simulink library "CryoDetLibCMB"  (R2016b)
settings: Solver=VariableStepAuto  StartTime=0.0  StopTime=10.0  RelTol=1e-3
undefined symbols (not defined in the file): A, B, C, D, Fadc, Fclk, PCIN, xlipgetpartsetting
libraries: xbsIndex_r4 x640, CryoDetLibCMB x81, CryoDetLib x2, simulink x1
(part 1 of 12)
settings Model: Creator=ssmith  LastModifiedBy=mdewart

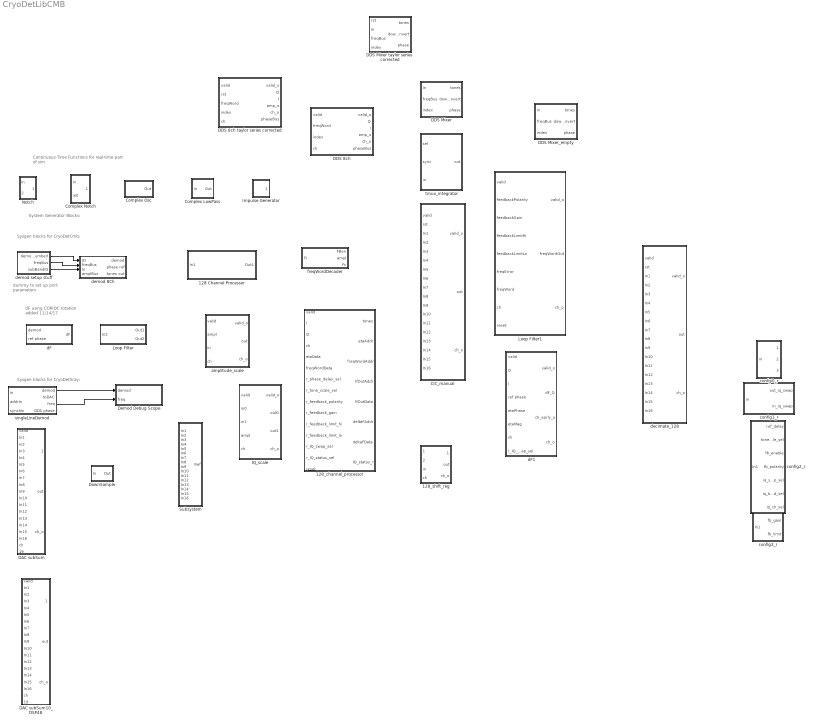
== system CryoDetLibCMB ==
  note: dummy to set up port parameters
  note: Sysgen blocks for CryoDetXray:
  note: Continuous-Time Functions
      | for real-time part of sim
  note: System Generator Blocks:
  note: Sysgen blocks for CryoDetCmb:
  note: dF using CORIDC rotation
      | added 11/14/17
  128 Channel Processor : Subsystem
  128_channel_processor : Subsystem
  128_shift_reg : Subsystem
  CIC_manual : Subsystem  mask{n_bit=30, b_pt=15}
      mask prompts: n_bit "Number of bits"; b_pt "Binary point"
  Complex LowPass : Subsystem  mask{num=0, den=0}
  Complex Notch : Subsystem  mask(Complex Notch Filter){Q=10, depth=1, Q1=10, depth1=1, Q2=10, depth2=1}
      mask help: Specify w0, Q, and notch depth (1 is max depth, 0 is no notch)
      mask init:
      | Q1 = Q
      | depth1 = depth
      | Q2 = Q
      | depth2 = depth
      mask TypeOptions Q1: Notch1/Q
      mask TypeOptions depth1: Notch1/depth
      mask TypeOptions Q2: Notch2/Q
      mask TypeOptions depth2: Notch2/depth
  Complex Osc : Subsystem  mask{Freq=40e6, Ampl=0.2}
  DAC subSum : Subsystem
  DAC subSum10_DSP48 : Subsystem  VariantControl=Variant1
  DDS 8ch : Subsystem
  DDS 8ch taylor series corrected : Subsystem
  DDS Mixer : Subsystem
  DDS Mixer taylor series corrected : Subsystem
  DDS Mixer_empty : Subsystem
  Demod Debug Scope : Subsystem
  DownSample : Subsystem
  IQ_scale : Subsystem
  Impulse Generator : Subsystem  mask(Impulse Generator){Impulse=0, width=0, Period=0, delay=0}
      mask help:
      | Generate an psuedo-impulse via a rectangular pulse of amplitude given impulse/width so time intagral is impulse
      | repeating at period given by parameter Period starting at time "delay"
  Loop Filter : Subsystem
  Loop Filter1 : Subsystem
  Notch : Subsystem  mask(Notch filter){Q=10, depth=1}
      mask help:
      | Continuous-time notch filter acting in input with input parameters:
      | w0	center frequency
      | Q	center frequency/bandwidth
      | depth	depth of notch: 0==> no notch, 1 ==> deep notch
  Subsystem : Subsystem
  amplitude_scale : Subsystem
  confgi0_r : Subsystem
  config1_r : Subsystem
  config2_r : Subsystem
  config3_r : Subsystem
  dF : Subsystem
  dF1 : Subsystem
  decimate_128 : Subsystem
  demod 8Ch : Subsystem
  demod setup stuff : Subsystem
  freqWordDecoder : Subsystem
  singleLineDemod : Subsystem
  tmux_integrator : Subsystem  mask{n_bit=18, b_pt=0}
      mask prompts: n_bit "Number of bits"; b_pt "Binary point"
  wires:
  singleLineDemod/3(freq) -> Demod Debug Scope/2(freq)
  singleLineDemod/1(demod) -> Demod Debug Scope/1(demod)
  demod setup stuff/3(subBandIQ) -> demod 8Ch/3(In)
  demod setup stuff/1(demod numberl) -> demod 8Ch/1(ID)
  demod setup stuff/2(freqBus) -> demod 8Ch/2(freqBus)

== system CryoDetLibCMB/128 Channel Processor ==
  note: 128 Channel Processor
      | Contains baeband tone generator
      | demodulator
      | resonator frequency error estimator
      | loop filter
  In1 : Inport
  128 Channel Demodulator : Subsystem
  Loop Filter : Subsystem
  dF : Subsystem
  Out1 : Outport
  wires:
  In1/1 -> 128 Channel Demodulator/1(in)
  dF/1(Out1) -> Loop Filter/1(In1)
  128 Channel Demodulator/1(demod) -> dF/1(demod in)
  Loop Filter/1(Out1) -> 128 Channel Demodulator/2(freqBus)
  128 Channel Demodulator/2(phase ref out) -> dF/2(phase ref in)

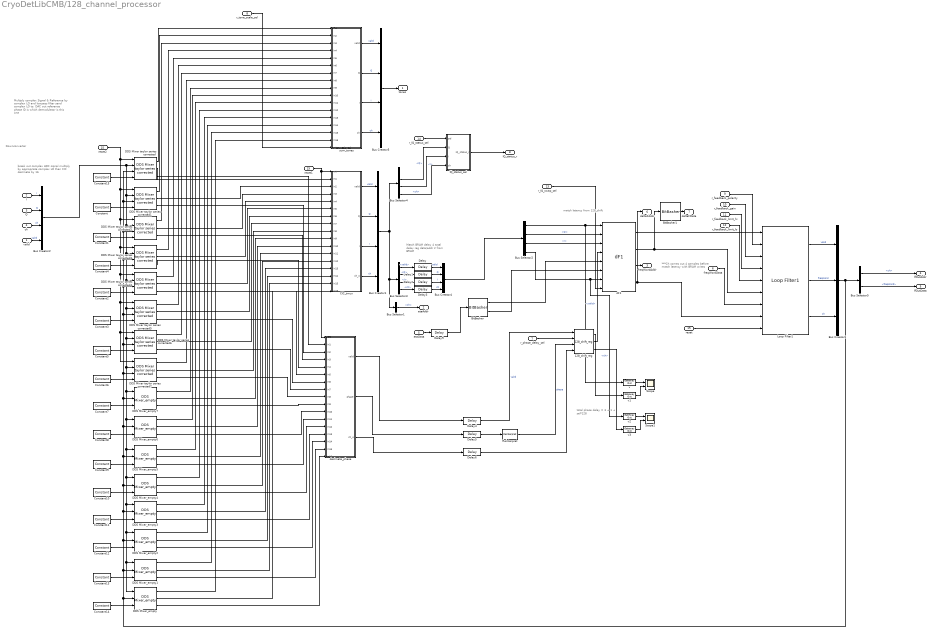
== system CryoDetLibCMB/128_channel_processor ==
  note: ***Ch comes out 4 samples before
      | match latency with BRAM writes
  note: total phase delay =
      | 3 + 1 + sel*128
  note: match latency from 128_shift
  note: Match BRAM delay
      | 4 total delay
      |    reg data/addr
      |    2 from BRAM
  note: break out complex ADC signal
      | multiply by appropriate complex LO
      | then CIC decimate by 16
  note: Multiply complex Signal & Reference
      | by complex LO and lowpass filter
      | send complex LO to:
      | 	DAC out
      | 	reference phase
      | ID is which demodulator is this one
  note: Downconverter
  valid : Inport
  I : Inport  Port=2
  Q : Inport  Port=3
  ch : Inport  Port=4
  etaData : Inport  Port=5
  freqWordData : Inport  Port=6
  r_phase_delay_sel : Inport  Port=7
  r_tone_scale_sel : Inport  Port=8
  r_feedback_polarity : Inport  Port=9
  r_feedback_gain : Inport  Port=10
  r_feedback_limit_hi : Inport  Port=11
  r_feedback_limit_lo : Inport  Port=12
  r_IQ_swap_sel : Inport  Port=13
  r_IQ_status_sel : Inport  Port=14
  reset : Inport  Port=15
  128_shift_reg : CryoDetLibCMB/128_shift_reg
  BitBasher : xbsIndex_r4/BitBasher  bitexpr=|  display_expr=off  sr_1=etaPhase  arith_type1="Signed  (2's comp)"  bin_pt1=15  sr_2=etaMag  arith_type2="Signed  (2's comp)"  bin_pt2=10  sr_3=3  arith_type3=Unsigned  bin_pt3=0  sr_4=4  arith_type4=Unsigned  bin_pt4=0  dbl_ovrd=off  block_type=bitbasher
      | etaPhase = {in[31:16]}
      | etaMag = {in[15:0]}
  BitBasher1 : xbsIndex_r4/BitBasher  bitexpr=deltaF = {8'b0, in[23:0]}  display_expr=off  sr_1=deltaF  arith_type1="Signed  (2's comp)"  bin_pt1=15  sr_2=etaMag  arith_type2="Signed  (2's comp)"  bin_pt2=10  sr_3=3  arith_type3=Unsigned  bin_pt3=0  sr_4=4  arith_type4=Unsigned  bin_pt4=0  dbl_ovrd=off  block_type=bitbasher
  Bus Creator{1..2,4..5} (4 alike) : BusCreator  Inputs=4
  Bus Creator3 : BusCreator  Inputs=3
  Bus Selector1 : BusSelector  OutputSignals=ch
  Bus Selector2 : BusSelector  OutputSignals=valid,Q,I,ch
  Bus Selector3 : BusSelector  OutputSignals=valid,Q,I,ch
  Bus Selector4 : BusSelector  OutputSignals=valid,Q,I,ch
  Bus Selector5 : BusSelector  OutputSignals=ch,freqWord
  CIC_tmux : Subsystem
  Constant : xbsIndex_r4/Constant  const=1  gui_display_data_type=Fixed-point  arith_type=Unsigned  n_bits=4  bin_pt=0  preci_type=Single  exp_width=8  frac_width=24  explicit_period=off  period=1  equ=P=C  opselect=C  inp2=PCIN>>17  opr=+  inp1=P  carry=CIN  dbl_ovrd=off  block_type=constant
  Constant1 : xbsIndex_r4/Constant  const=2  gui_display_data_type=Fixed-point  arith_type=Unsigned  n_bits=4  bin_pt=0  preci_type=Single  exp_width=8  frac_width=24  explicit_period=off  period=1  equ=P=C  opselect=C  inp2=PCIN>>17  opr=+  inp1=P  carry=CIN  dbl_ovrd=off  block_type=constant
  Constant10 : xbsIndex_r4/Constant  const=11  gui_display_data_type=Fixed-point  arith_type=Unsigned  n_bits=4  bin_pt=0  preci_type=Single  exp_width=8  frac_width=24  explicit_period=off  period=1  equ=P=C  opselect=C  inp2=PCIN>>17  opr=+  inp1=P  carry=CIN  dbl_ovrd=off  block_type=constant
  Constant11 : xbsIndex_r4/Constant  const=12  gui_display_data_type=Fixed-point  arith_type=Unsigned  n_bits=4  bin_pt=0  preci_type=Single  exp_width=8  frac_width=24  explicit_period=off  period=1  equ=P=C  opselect=C  inp2=PCIN>>17  opr=+  inp1=P  carry=CIN  dbl_ovrd=off  block_type=constant
  Constant12 : xbsIndex_r4/Constant  const=13  gui_display_data_type=Fixed-point  arith_type=Unsigned  n_bits=4  bin_pt=0  preci_type=Single  exp_width=8  frac_width=24  explicit_period=off  period=1  equ=P=C  opselect=C  inp2=PCIN>>17  opr=+  inp1=P  carry=CIN  dbl_ovrd=off  block_type=constant
  Constant13 : xbsIndex_r4/Constant  const=14  gui_display_data_type=Fixed-point  arith_type=Unsigned  n_bits=4  bin_pt=0  preci_type=Single  exp_width=8  frac_width=24  explicit_period=off  period=1  equ=P=C  opselect=C  inp2=PCIN>>17  opr=+  inp1=P  carry=CIN  dbl_ovrd=off  block_type=constant
  Constant14 : xbsIndex_r4/Constant  const=15  gui_display_data_type=Fixed-point  arith_type=Unsigned  n_bits=4  bin_pt=0  preci_type=Single  exp_width=8  frac_width=24  explicit_period=off  period=1  equ=P=C  opselect=C  inp2=PCIN>>17  opr=+  inp1=P  carry=CIN  dbl_ovrd=off  block_type=constant
  Constant15 : xbsIndex_r4/Constant  const=0  gui_display_data_type=Fixed-point  arith_type=Unsigned  n_bits=4  bin_pt=0  preci_type=Single  exp_width=8  frac_width=24  explicit_period=off  period=1  equ=P=C  opselect=C  inp2=PCIN>>17  opr=+  inp1=P  carry=CIN  dbl_ovrd=off  block_type=constant
  Constant2 : xbsIndex_r4/Constant  const=4  gui_display_data_type=Fixed-point  arith_type=Unsigned  n_bits=4  bin_pt=0  preci_type=Single  exp_width=8  frac_width=24  explicit_period=off  period=1  equ=P=C  opselect=C  inp2=PCIN>>17  opr=+  inp1=P  carry=CIN  dbl_ovrd=off  block_type=constant
  Constant3 : xbsIndex_r4/Constant  const=5  gui_display_data_type=Fixed-point  arith_type=Unsigned  n_bits=4  bin_pt=0  preci_type=Single  exp_width=8  frac_width=24  explicit_period=off  period=1  equ=P=C  opselect=C  inp2=PCIN>>17  opr=+  inp1=P  carry=CIN  dbl_ovrd=off  block_type=constant
  Constant4 : xbsIndex_r4/Constant  const=3  gui_display_data_type=Fixed-point  arith_type=Unsigned  n_bits=4  bin_pt=0  preci_type=Single  exp_width=8  frac_width=24  explicit_period=off  period=1  equ=P=C  opselect=C  inp2=PCIN>>17  opr=+  inp1=P  carry=CIN  dbl_ovrd=off  block_type=constant
  Constant5 : xbsIndex_r4/Constant  const=6  gui_display_data_type=Fixed-point  arith_type=Unsigned  n_bits=4  bin_pt=0  preci_type=Single  exp_width=8  frac_width=24  explicit_period=off  period=1  equ=P=C  opselect=C  inp2=PCIN>>17  opr=+  inp1=P  carry=CIN  dbl_ovrd=off  block_type=constant
  Constant6 : xbsIndex_r4/Constant  const=7  gui_display_data_type=Fixed-point  arith_type=Unsigned  n_bits=4  bin_pt=0  preci_type=Single  exp_width=8  frac_width=24  explicit_period=off  period=1  equ=P=C  opselect=C  inp2=PCIN>>17  opr=+  inp1=P  carry=CIN  dbl_ovrd=off  block_type=constant
  Constant7 : xbsIndex_r4/Constant  const=8  gui_display_data_type=Fixed-point  arith_type=Unsigned  n_bits=4  bin_pt=0  preci_type=Single  exp_width=8  frac_width=24  explicit_period=off  period=1  equ=P=C  opselect=C  inp2=PCIN>>17  opr=+  inp1=P  carry=CIN  dbl_ovrd=off  block_type=constant
  Constant8 : xbsIndex_r4/Constant  const=9  gui_display_data_type=Fixed-point  arith_type=Unsigned  n_bits=4  bin_pt=0  preci_type=Single  exp_width=8  frac_width=24  explicit_period=off  period=1  equ=P=C  opselect=C  inp2=PCIN>>17  opr=+  inp1=P  carry=CIN  dbl_ovrd=off  block_type=constant
  Constant9 : xbsIndex_r4/Constant  const=10  gui_display_data_type=Fixed-point  arith_type=Unsigned  n_bits=4  bin_pt=0  preci_type=Single  exp_width=8  frac_width=24  explicit_period=off  period=1  equ=P=C  opselect=C  inp2=PCIN>>17  opr=+  inp1=P  carry=CIN  dbl_ovrd=off  block_type=constant
  DDS Mixer taylor series corrected : CryoDetLibCMB/DDS Mixer taylor series corrected
      link override DDS 8ch taylor series corrected/BitBasher5: bitexpr=phase = {in[23:8]}  display_expr=off  sr_1=phase  arith_type1="Signed  (2's comp)"  bin_pt1=15  sr_2=amp  arith_type2=Unsigned  bin_pt2=0  sr_3=3  arith_type3=Unsigned  bin_pt3=0  sr_4=4  arith_type4=Unsigned  bin_pt4=0  dbl_ovrd=off
      link override DDS 8ch taylor series corrected/BitBasher5: infoedit=Allows extraction, concatenation and augmentation of bits
  DDS Mixer taylor series corrected{1..7} (7 alike) : CryoDetLibCMB/DDS Mixer taylor series corrected
  DDS Mixer_empty{,1..7} (8 alike) : CryoDetLibCMB/DDS Mixer_empty
  Delay{,1..3} (4 alike) : xbsIndex_r4/Delay  rst=off  infoeditControl=Selection of Reset will increase slice count due to use of real FFs and instead of SRLs  en=off  latency=5  reg_retiming=off  dbl_ovrd=off  block_type=delay
  Delay4 : xbsIndex_r4/Delay  rst=off  infoeditControl=Selection of Reset will increase slice count due to use of real FFs and instead of SRLs  en=off  latency=12  reg_retiming=off  dbl_ovrd=off  block_type=delay
  Delay5 : xbsIndex_r4/Delay  rst=off  infoeditControl=Selection of Reset will increase slice count due to use of real FFs and instead of SRLs  en=off  latency=12  reg_retiming=off  dbl_ovrd=off  block_type=delay
  Delay6 : xbsIndex_r4/Delay  rst=off  infoeditControl=Selection of Reset will increase slice count due to use of real FFs and instead of SRLs  en=off  latency=12  reg_retiming=off  dbl_ovrd=off  block_type=delay
  Delay9 : xbsIndex_r4/Delay  rst=off  infoeditControl=Selection of Reset will increase slice count due to use of real FFs and instead of SRLs  en=off  latency=1  reg_retiming=off  dbl_ovrd=off  block_type=delay
  IQ_status_sel : Subsystem
  Loop Filter1 : CryoDetLibCMB/Loop Filter1
  Reinterpret : xbsIndex_r4/Reinterpret  force_arith_type=on  arith_type="Signed  (2's comp)"  force_bin_pt=on  bin_pt=15  block_type=reinterpret
  Scope : Scope  NumInputPorts=2
  Scope1 : Scope  NumInputPorts=2
  dF1 : CryoDetLibCMB/dF1
  decimate_phase : Subsystem
  reset1 : InportShadow  Port=15
  reset2 : InportShadow  Port=15
  sum_tones : Subsystem
  v{,1..3} (4 alike) : xbsIndex_r4/Gateway Out  inherit_from_input=off  hdl_port=off  rows=1  columns=1  UseAsDAC=off  DACChannel='1'  interface=None  automatic_assignment=on  address_offset=hex2dec('00')  intf_name=''  intf_description=''  timing_constraint=None  locs_specified=off  LOCs={}  io_standard={}  block_type=gatewayout
  tones : Outport
  etaAddr : Outport  Port=2
  freqWordAddr : Outport  Port=3
  lfOutAddr : Outport  Port=4
  lfOutData : Outport  Port=5
  deltaFAddr : Outport  Port=6
  deltaFData : Outport  Port=7
  IQ_status_r : Outport  Port=8
  wires:
  reset2/1 -> DDS Mixer taylor series corrected2/1, DDS Mixer taylor series corrected3/1, DDS Mixer taylor series corrected4/1, DDS Mixer taylor series corrected5/1, DDS Mixer taylor series corrected6/1, DDS Mixer taylor series corrected7/1, DDS Mixer taylor series corrected1/1, DDS Mixer taylor series corrected/1
  Bus Creator3/1 -> DDS Mixer_empty/2, DDS Mixer_empty1/2, DDS Mixer_empty2/2, DDS Mixer_empty3/2, DDS Mixer_empty4/2, DDS Mixer_empty5/2, DDS Mixer taylor series corrected/3, DDS Mixer taylor series corrected1/3, DDS Mixer taylor series corrected2/3, DDS Mixer taylor series corrected3/3, DDS Mixer taylor series corrected4/3, DDS Mixer taylor series corrected5/3, DDS Mixer taylor series corrected6/3, DDS Mixer taylor series corrected7/3, DDS Mixer_empty7/2, DDS Mixer_empty6/2, Bus Selector5/1
  Constant6/1 -> DDS Mixer taylor series corrected7/4
  Constant5/1 -> DDS Mixer taylor series corrected6/4
  Constant3/1 -> DDS Mixer taylor series corrected5/4
  Constant2/1 -> DDS Mixer taylor series corrected4/4
  Constant4/1 -> DDS Mixer taylor series corrected3/4
  Constant1/1 -> DDS Mixer taylor series corrected2/4
  Constant/1 -> DDS Mixer taylor series corrected1/4
  Constant15/1 -> DDS Mixer taylor series corrected/4
  reset1/1 -> CIC_tmux/1(rst), decimate_phase/1(rst)
  Delay6/1 -> 128_shift_reg/4
  Delay9/1 -> BitBasher/1
  IQ_status_sel/1(IQ_status_r) -> IQ_status_r/1
  r_IQ_status_sel/1 -> IQ_status_sel/1(sel)
  Bus Selector4/4 -> IQ_status_sel/4(ch)  "<ch>"
  Bus Selector4/3 -> IQ_status_sel/3(I)  "<I>"
  Bus Selector4/2 -> IQ_status_sel/2(Q)  "<Q>"
  r_IQ_swap_sel/1 -> dF1/8
  128_shift_reg/3 -> v3/1
  v3/1 -> Scope1/2
  v2/1 -> Scope1/1
  128_shift_reg/1 -> v1/1
  v1/1 -> Scope/2
  v/1 -> Scope/1
  DDS Mixer taylor series corrected/2 -> CIC_tmux/2(In1)
  DDS Mixer taylor series corrected1/2 -> CIC_tmux/3(In2)
  DDS Mixer taylor series corrected2/2 -> CIC_tmux/4(In3)
  DDS Mixer taylor series corrected3/2 -> CIC_tmux/5(In4)
  DDS Mixer taylor series corrected4/2 -> CIC_tmux/6(In5)
  DDS Mixer taylor series corrected5/2 -> CIC_tmux/7(In6)
  DDS Mixer taylor series corrected6/2 -> CIC_tmux/8(In7)
  DDS Mixer taylor series corrected7/2 -> CIC_tmux/9(In8)
  DDS Mixer_empty7/2 -> CIC_tmux/10(In9)
  DDS Mixer_empty6/2 -> CIC_tmux/11(In10)
  DDS Mixer_empty5/2 -> CIC_tmux/12(In11)
  DDS Mixer_empty4/2 -> CIC_tmux/13(In12)
  DDS Mixer_empty3/2 -> CIC_tmux/14(In13)
  DDS Mixer_empty2/2 -> CIC_tmux/15(In14)
  DDS Mixer_empty1/2 -> CIC_tmux/16(In15)
  DDS Mixer_empty/2 -> CIC_tmux/17(In16)
  Bus Creator2/1 -> DDS Mixer_empty5/1, DDS Mixer_empty4/1, DDS Mixer_empty3/1, DDS Mixer_empty2/1, DDS Mixer_empty1/1, DDS Mixer_empty/1, DDS Mixer_empty6/1, DDS Mixer_empty7/1, DDS Mixer taylor series corrected7/2, DDS Mixer taylor series corrected6/2, DDS Mixer taylor series corrected5/2, DDS Mixer taylor series corrected4/2, DDS Mixer taylor series corrected3/2, DDS Mixer taylor series corrected2/2, DDS Mixer taylor series corrected1/2, DDS Mixer taylor series corrected/2
  Constant14/1 -> DDS Mixer_empty/3
  Constant13/1 -> DDS Mixer_empty1/3
  Constant12/1 -> DDS Mixer_empty2/3
  Constant11/1 -> DDS Mixer_empty3/3
  Constant10/1 -> DDS Mixer_empty4/3
  Constant9/1 -> DDS Mixer_empty5/3
  Constant8/1 -> DDS Mixer_empty6/3
  Constant7/1 -> DDS Mixer_empty7/3
  DDS Mixer taylor series corrected/1 -> sum_tones/1(In1)
  DDS Mixer taylor series corrected1/1 -> sum_tones/2(In2)
  DDS Mixer taylor series corrected2/1 -> sum_tones/3(In3)
  DDS Mixer taylor series corrected3/1 -> sum_tones/4(In4)
  DDS Mixer taylor series corrected4/1 -> sum_tones/5(In5)
  DDS Mixer taylor series corrected5/1 -> sum_tones/6(In6)
  DDS Mixer taylor series corrected6/1 -> sum_tones/7(In7)
  DDS Mixer taylor series corrected7/1 -> sum_tones/8(In8)
  DDS Mixer_empty7/1 -> sum_tones/9(In9)
  DDS Mixer_empty6/1 -> sum_tones/10(In10)
  DDS Mixer_empty5/1 -> sum_tones/11(In11)
  DDS Mixer_empty4/1 -> sum_tones/12(In12)
  DDS Mixer_empty3/1 -> sum_tones/13(In13)
  DDS Mixer_empty2/1 -> sum_tones/14(In14)
  DDS Mixer_empty1/1 -> sum_tones/15(In15)
  DDS Mixer_empty/1 -> sum_tones/16(In16)
  I/1 -> Bus Creator2/1  "I"
  Q/1 -> Bus Creator2/2  "Q"
  ch/1 -> Bus Creator2/3  "ch"
  valid/1 -> Bus Creator2/4  "valid"
  Bus Creator1/1 -> Bus Selector4/1, Bus Selector3/1, Bus Selector1/1
  Bus Selector1/1 -> etaAddr/1  "<ch>"
  Delay/1 -> Bus Creator4/1  "valid"
  Delay1/1 -> Bus Creator4/2  "Q"
  Delay2/1 -> Bus Creator4/3  "I"
  Delay3/1 -> Bus Creator4/4  "ch"
  etaData/1 -> Delay9/1
  Bus Creator4/1 -> Bus Selector2/1
  BitBasher1/1 -> deltaFData/1
  CIC_tmux/1(valid) -> Bus Creator1/1  "valid"
  CIC_tmux/2(Q) -> Bus Creator1/2  "Q"
  CIC_tmux/3(I) -> Bus Creator1/3  "I"
  CIC_tmux/4(ch_o) -> Bus Creator1/4  "ch"
  Bus Selector3/1 -> Delay/1  "<valid>"
  Bus Selector3/2 -> Delay1/1  "<Q>"
  Bus Selector3/3 -> Delay2/1  "<I>"
  Bus Selector3/4 -> Delay3/1  "<ch>"
  sum_tones/3(I) -> Bus Creator5/3  "I"
  sum_tones/2(Q) -> Bus Creator5/2  "Q"
  sum_tones/4(ch) -> Bus Creator5/4  "ch"
  sum_tones/1(valid) -> Bus Creator5/1  "valid"
  Bus Creator5/1 -> tones/1
  Bus Selector2/1 -> dF1/1, v/1  "<valid>"
  Bus Selector2/2 -> dF1/2  "<Q>"
  Bus Selector2/3 -> dF1/3  "<I>"
  Bus Selector2/4 -> dF1/7, v2/1  "<ch>"
  128_shift_reg/2 -> dF1/4
  dF1/1 -> Loop Filter1/1
  Loop Filter1/1 -> Bus Creator3/1  "valid"
  Bus Selector5/2 -> lfOutData/1  "<freqWord>"
  Bus Selector5/1 -> lfOutAddr/1  "<ch>"
  r_phase_delay_sel/1 -> 128_shift_reg/2
  r_feedback_limit_hi/1 -> Loop Filter1/4
  r_feedback_gain/1 -> Loop Filter1/3
  r_feedback_polarity/1 -> Loop Filter1/2
  r_tone_scale_sel/1 -> sum_tones/17(r_tone_scale_sel)
  Loop Filter1/2 -> Bus Creator3/2  "freqWord"
  Loop Filter1/3 -> Bus Creator3/3  "ch"
  DDS Mixer_empty/3 -> decimate_phase/17(In16)
  DDS Mixer_empty1/3 -> decimate_phase/16(In15)
  DDS Mixer_empty2/3 -> decimate_phase/15(In14)
  DDS Mixer_empty3/3 -> decimate_phase/14(In13)
  DDS Mixer_empty4/3 -> decimate_phase/13(In12)
  DDS Mixer_empty5/3 -> decimate_phase/12(In11)
  DDS Mixer_empty6/3 -> decimate_phase/11(In10)
  DDS Mixer_empty7/3 -> decimate_phase/10(In9)
  DDS Mixer taylor series corrected7/3 -> decimate_phase/9(In8)
  DDS Mixer taylor series corrected6/3 -> decimate_phase/8(In7)
  DDS Mixer taylor series corrected5/3 -> decimate_phase/7(In6)
  DDS Mixer taylor series corrected4/3 -> decimate_phase/6(In5)
  DDS Mixer taylor series corrected3/3 -> decimate_phase/5(In4)
  DDS Mixer taylor series corrected2/3 -> decimate_phase/4(In3)
  DDS Mixer taylor series corrected1/3 -> decimate_phase/3(In2)
  DDS Mixer taylor series corrected/3 -> decimate_phase/2(In1)
  decimate_phase/1(valid) -> Delay4/1
  decimate_phase/3(ch_o) -> Delay6/1
  decimate_phase/2(phase) -> Delay5/1
  BitBasher/1 -> dF1/5
  BitBasher/2 -> dF1/6
  Delay5/1 -> Reinterpret/1
  Delay4/1 -> 128_shift_reg/1  "valid"
  Reinterpret/1 -> 128_shift_reg/3  "phase"
  reset/1 -> Loop Filter1/9
  dF1/3 -> freqWordAddr/1
  dF1/2 -> Loop Filter1/6, BitBasher1/1
  r_feedback_limit_lo/1 -> Loop Filter1/5
  freqWordData/1 -> Loop Filter1/7
  dF1/4 -> Loop Filter1/8, deltaFAddr/1

== system CryoDetLibCMB/128_shift_reg ==
  note: Ch, valid only delayed to match MUX
  valid_i : Inport
  sel_3_0 : Inport  Port=2
  in : Inport  Port=3
  ch : Inport  Port=4
  AddSub : xbsIndex_r4/AddSub  mode=Subtraction  use_carryin=off  use_carryout=off  en=off  latency=3  precision=User Defined  arith_type="Signed  (2's comp)"  n_bits=16  bin_pt=15  quantization=Truncate  overflow=Wrap  use_behavioral_HDL=off  hw_selection=Fabric  pipelined=off  dbl_ovrd=off  block_type=addsub
  Delay{1..6,8} (7 alike) : xbsIndex_r4/Delay  rst=off  infoeditControl=Selection of Reset will increase slice count due to use of real FFs and instead of SRLs  en=off  latency=128  reg_retiming=off  dbl_ovrd=off  block_type=delay
  Delay7 : xbsIndex_r4/Delay  rst=off  infoeditControl=Selection of Reset will increase slice count due to use of real FFs and instead of SRLs  en=off  latency=4  reg_retiming=off  dbl_ovrd=off  block_type=delay
  Delay9 : xbsIndex_r4/Delay  rst=off  infoeditControl=Selection of Reset will increase slice count due to use of real FFs and instead of SRLs  en=off  latency=4  reg_retiming=off  dbl_ovrd=off  block_type=delay
  Mux : xbsIndex_r4/Mux  inputs=8  en=off  latency=1  precision=Full  arith_type=Unsigned  n_bits=16  bin_pt=14  quantization=Truncate  overflow=Wrap  dbl_ovrd=off  block_type=mux
  Register2 : xbsIndex_r4/Register  init=0  rst=off  en=off  dbl_ovrd=off  block_type=register
  valid_o : Outport
  out : Outport  Port=2
  ch_o : Outport  Port=3
  wires:
  Mux/1 -> AddSub/2
  Register2/1 -> AddSub/1
  in/1 -> Delay5/1, Mux/2, Register2/1
  AddSub/1 -> out/1
  Delay1/1 -> Mux/6, Delay4/1
  Delay8/1 -> Mux/4, Delay2/1
  Delay5/1 -> Mux/3, Delay8/1
  sel_3_0/1 -> Mux/1
  Delay6/1 -> Mux/9
  Delay4/1 -> Mux/7, Delay3/1
  Delay2/1 -> Mux/5, Delay1/1
  Delay3/1 -> Mux/8, Delay6/1
  ch/1 -> Delay7/1
  Delay7/1 -> ch_o/1
  valid_i/1 -> Delay9/1
  Delay9/1 -> valid_o/1

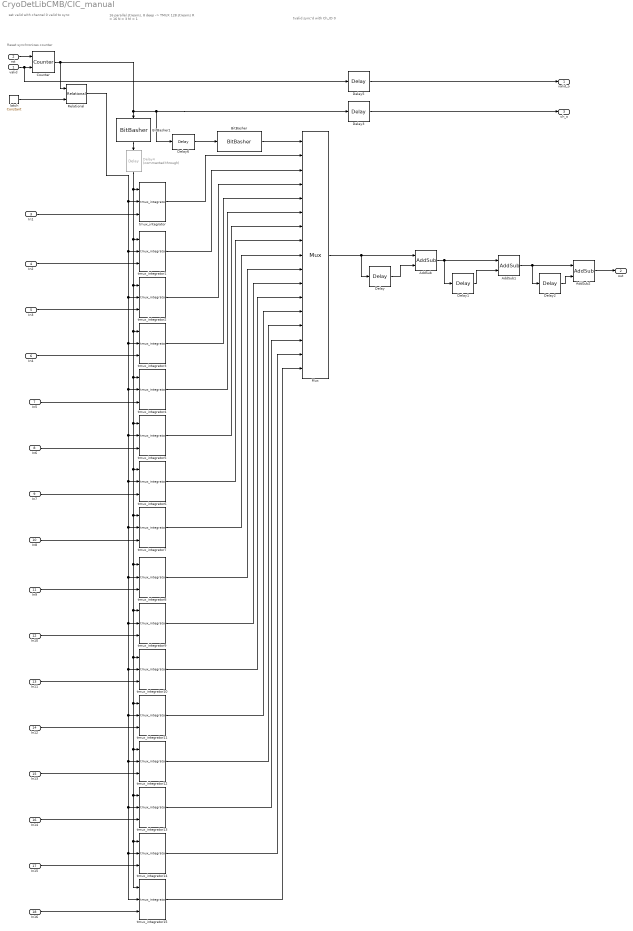
== system CryoDetLibCMB/CIC_manual ==
  note: tvalid sync'd with Ch_ID 0
  note: set valid with channel 0 valid to sync
  note: Reset synchronizes counter
  note: 16 parallel streams, 8 deep -> TMUX 128 streams
      | R = 16
      | N = 3
      | M = 1
  valid : Inport
  rst : Inport  Port=2
  In1 : Inport  Port=3
  In2 : Inport  Port=4
  In3 : Inport  Port=5
  In4 : Inport  Port=6
  In5 : Inport  Port=7
  In6 : Inport  Port=8
  In7 : Inport  Port=9
  In8 : Inport  Port=10
  In9 : Inport  Port=11
  In10 : Inport  Port=12
  In11 : Inport  Port=13
  In12 : Inport  Port=14
  In13 : Inport  Port=15
  In14 : Inport  Port=16
  In15 : Inport  Port=17
  In16 : Inport  Port=18
  AddSub : xbsIndex_r4/AddSub  mode=Subtraction  use_carryin=off  use_carryout=off  en=off  latency=3  precision=User Defined  arith_type="Signed  (2's comp)"  n_bits=n_bit  bin_pt=b_pt  quantization=Truncate  overflow=Wrap  use_behavioral_HDL=on  hw_selection=Fabric  pipelined=off  dbl_ovrd=off  block_type=addsub
  AddSub1 : xbsIndex_r4/AddSub  mode=Subtraction  use_carryin=off  use_carryout=off  en=off  latency=3  precision=User Defined  arith_type="Signed  (2's comp)"  n_bits=n_bit  bin_pt=b_pt  quantization=Truncate  overflow=Wrap  use_behavioral_HDL=on  hw_selection=Fabric  pipelined=off  dbl_ovrd=off  block_type=addsub
  AddSub2 : xbsIndex_r4/AddSub  mode=Subtraction  use_carryin=off  use_carryout=off  en=off  latency=3  precision=User Defined  arith_type="Signed  (2's comp)"  n_bits=n_bit  bin_pt=b_pt  quantization=Truncate  overflow=Wrap  use_behavioral_HDL=on  hw_selection=Fabric  pipelined=off  dbl_ovrd=off  block_type=addsub
  BitBasher : xbsIndex_r4/BitBasher  bitexpr=sel = {cnt[3:0]}  display_expr=on  sr_1=sel  arith_type1=Unsigned  bin_pt1=0  sr_2=2  arith_type2=Unsigned  bin_pt2=0  sr_3=3  arith_type3=Unsigned  bin_pt3=0  sr_4=4  arith_type4=Unsigned  bin_pt4=0  dbl_ovrd=off  block_type=bitbasher
  BitBasher1 : xbsIndex_r4/BitBasher  bitexpr=sel = {cnt[6:4]}  display_expr=on  sr_1=sel  arith_type1=Unsigned  bin_pt1=0  sr_2=2  arith_type2=Unsigned  bin_pt2=0  sr_3=3  arith_type3=Unsigned  bin_pt3=0  sr_4=4  arith_type4=Unsigned  bin_pt4=0  dbl_ovrd=off  block_type=bitbasher
  Counter : xbsIndex_r4/Counter  cnt_type=Free Running  cnt_to=Inf  operation=Up  start_count=0  cnt_by_val=1  arith_type=Unsigned  n_bits=7  bin_pt=0  load_pin=off  rst=on  en=on  explicit_period=on  period=2/Fadc  use_behavioral_HDL=off  implementation=Fabric  dbl_ovrd=off  block_type=counter
  Delay : xbsIndex_r4/Delay  rst=off  infoeditControl=Selection of Reset will increase slice count due to use of real FFs and instead of SRLs  en=off  latency=128  reg_retiming=on  dbl_ovrd=off  block_type=delay
  Delay1 : xbsIndex_r4/Delay  rst=off  infoeditControl=Selection of Reset will increase slice count due to use of real FFs and instead of SRLs  en=off  latency=128  reg_retiming=on  dbl_ovrd=off  block_type=delay
  Delay2 : xbsIndex_r4/Delay  rst=off  infoeditControl=Selection of Reset will increase slice count due to use of real FFs and instead of SRLs  en=off  latency=128  reg_retiming=on  dbl_ovrd=off  block_type=delay
  Delay3 : xbsIndex_r4/Delay  rst=off  infoeditControl=Selection of Reset will increase slice count due to use of real FFs and instead of SRLs  en=off  latency=11  reg_retiming=on  dbl_ovrd=off  block_type=delay
  Delay4 : xbsIndex_r4/Delay  Commented=through  rst=off  infoeditControl=Selection of Reset will increase slice count due to use of real FFs and instead of SRLs  en=off  latency=1  reg_retiming=on  dbl_ovrd=off  block_type=delay
  Delay5 : xbsIndex_r4/Delay  rst=off  infoeditControl=Selection of Reset will increase slice count due to use of real FFs and instead of SRLs  en=off  latency=11  reg_retiming=on  dbl_ovrd=off  block_type=delay
  Delay6 : xbsIndex_r4/Delay  rst=off  infoeditControl=Selection of Reset will increase slice count due to use of real FFs and instead of SRLs  en=off  latency=1  reg_retiming=on  dbl_ovrd=off  block_type=delay
  Mux : xbsIndex_r4/Mux  inputs=16  en=off  latency=1  precision=Full  arith_type=Unsigned  n_bits=16  bin_pt=14  quantization=Truncate  overflow=Wrap  dbl_ovrd=off  block_type=mux
  Relational : xbsIndex_r4/Relational  mode=a=b  op_type=Bool  en=off  latency=1  dbl_ovrd=off  block_type=relational
  latch : xbsIndex_r4/Constant  const=0  gui_display_data_type=Fixed-point  arith_type=Unsigned  n_bits=7  bin_pt=0  preci_type=Single  exp_width=8  frac_width=24  explicit_period=on  period=2/Fadc  equ=P=C  opselect=C  inp2=PCIN>>17  opr=+  inp1=P  carry=CIN  dbl_ovrd=off  block_type=constant
  tmux_integrator{,1..15} (16 alike) : CryoDetLibCMB/tmux_integrator  n_bit=n_bit  b_pt=b_pt
  valid_o : Outport
  out : Outport  Port=2
  ch_o : Outport  Port=3
  wires:
  rst/1 -> Counter/1
  Delay6/1 -> BitBasher/1
  Delay2/1 -> AddSub2/2
  Delay1/1 -> AddSub1/2
  Delay/1 -> AddSub/2
  latch/1 -> Relational/2
  Relational/1 -> tmux_integrator/2, tmux_integrator1/2, tmux_integrator2/2, tmux_integrator3/2, tmux_integrator4/2, tmux_integrator5/2, tmux_integrator6/2, tmux_integrator7/2, tmux_integrator8/2, tmux_integrator9/2, tmux_integrator10/2, tmux_integrator11/2, tmux_integrator12/2, tmux_integrator13/2, tmux_integrator15/2, tmux_integrator14/2
  BitBasher/1 -> Mux/1
  tmux_integrator/1 -> Mux/2
  tmux_integrator1/1 -> Mux/3
  tmux_integrator2/1 -> Mux/4
  tmux_integrator4/1 -> Mux/6
  tmux_integrator5/1 -> Mux/7
  tmux_integrator6/1 -> Mux/8
  tmux_integrator7/1 -> Mux/9
  tmux_integrator8/1 -> Mux/10
  tmux_integrator9/1 -> Mux/11
  tmux_integrator10/1 -> Mux/12
  tmux_integrator11/1 -> Mux/13
  tmux_integrator12/1 -> Mux/14
  tmux_integrator13/1 -> Mux/15
  tmux_integrator14/1 -> Mux/16
  tmux_integrator15/1 -> Mux/17
  In1/1 -> tmux_integrator/3
  In2/1 -> tmux_integrator1/3
  In3/1 -> tmux_integrator2/3
  In4/1 -> tmux_integrator3/3
  In5/1 -> tmux_integrator4/3
  In6/1 -> tmux_integrator5/3
  In7/1 -> tmux_integrator6/3
  In8/1 -> tmux_integrator7/3
  In9/1 -> tmux_integrator8/3
  In10/1 -> tmux_integrator9/3
  In11/1 -> tmux_integrator10/3
  In12/1 -> tmux_integrator11/3
  In13/1 -> tmux_integrator12/3
  In14/1 -> tmux_integrator13/3
  In15/1 -> tmux_integrator14/3
  In16/1 -> tmux_integrator15/3
  Mux/1 -> AddSub/1, Delay/1
  AddSub2/1 -> out/1
  tmux_integrator3/1 -> Mux/5
  BitBasher1/1 -> Delay4/1
  AddSub/1 -> AddSub1/1, Delay1/1
  AddSub1/1 -> AddSub2/1, Delay2/1
  valid/1 -> Delay5/1, Counter/2
  Delay3/1 -> ch_o/1
  Delay4/1 -> tmux_integrator/1, tmux_integrator1/1, tmux_integrator2/1, tmux_integrator3/1, tmux_integrator4/1, tmux_integrator5/1, tmux_integrator6/1, tmux_integrator7/1, tmux_integrator8/1, tmux_integrator9/1, tmux_integrator10/1, tmux_integrator11/1, tmux_integrator12/1, tmux_integrator13/1, tmux_integrator15/1, tmux_integrator14/1
  Counter/1 -> Relational/1, Delay6/1, Delay3/1, BitBasher1/1
  Delay5/1 -> valid_o/1

== system CryoDetLibCMB/Complex LowPass ==
  note: Apply continuous-time transfer function given by num/den to complex continuous-time signal
  In : Inport
  Complex to Real-Imag : ComplexToRealImag
  Real-Imag to Complex : RealImagToComplex
  Transfer Fcn : TransferFcn  Numerator=num  Denominator=den
  Transfer Fcn1 : TransferFcn  Numerator=num  Denominator=den
  Out : Outport
  wires:
  Complex to Real-Imag/2 -> Transfer Fcn1/1
  Transfer Fcn1/1 -> Real-Imag to Complex/2
  In/1 -> Complex to Real-Imag/1
  Real-Imag to Complex/1 -> Out/1
  Transfer Fcn/1 -> Real-Imag to Complex/1
  Complex to Real-Imag/1 -> Transfer Fcn/1

== system CryoDetLibCMB/Complex Notch ==
  In : Inport
  w0 : Inport  Port=2
  Complex to Real-Imag : ComplexToRealImag
  Notch1 : CryoDetLib/Notch  Q=Q1  depth=depth1
  Notch2 : CryoDetLib/Notch  Q=Q2  depth=depth2
  Real-Imag to Complex : RealImagToComplex
  Out : Outport
  wires:
  Complex to Real-Imag/2 -> Notch2/1
  Notch2/1 -> Real-Imag to Complex/2
  In/1 -> Complex to Real-Imag/1
  Real-Imag to Complex/1 -> Out/1
  Notch1/1 -> Real-Imag to Complex/1
  w0/1 -> Notch2/2, Notch1/2
  Complex to Real-Imag/1 -> Notch1/1

== system CryoDetLibCMB/Complex Osc ==
  Cosine : Sin  Amplitude=Ampl  Frequency=2*pi*Freq  Phase=pi/2  SampleTime=0
  Real-Imag to Complex : RealImagToComplex
  Sine : Sin  Amplitude=Ampl  Frequency=2*pi*Freq  SampleTime=0
  Out : Outport
  wires:
  Real-Imag to Complex/1 -> Out/1
  Cosine/1 -> Real-Imag to Complex/1
  Sine/1 -> Real-Imag to Complex/2

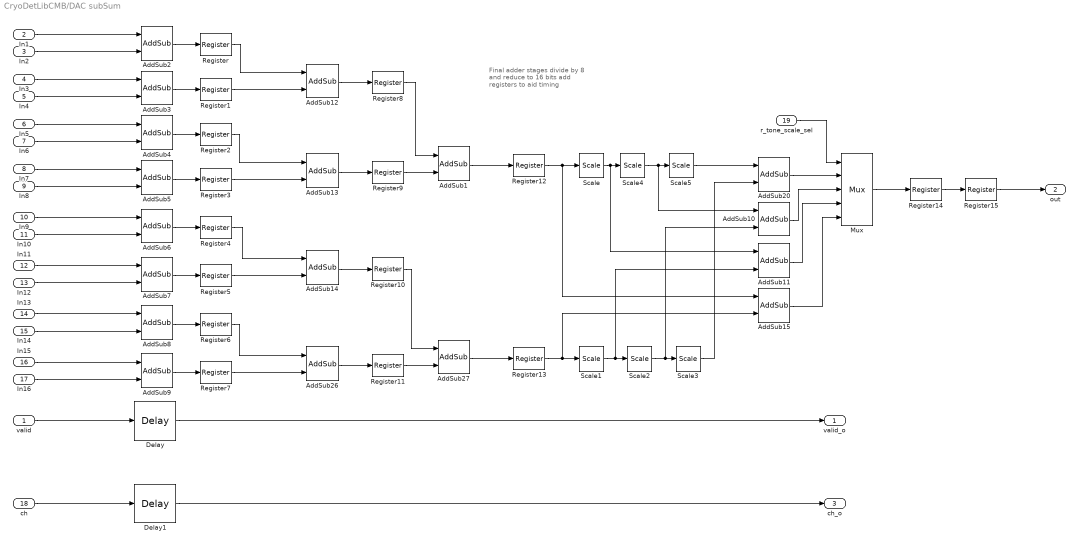
== system CryoDetLibCMB/DAC subSum ==
  note: Final adder stages
      | divide by 8
      | and reduce to 16 bits
      | add registers to aid timing
  valid : Inport
  In1 : Inport  Port=2
  In2 : Inport  Port=3
  In3 : Inport  Port=4
  In4 : Inport  Port=5
  In5 : Inport  Port=6
  In6 : Inport  Port=7
  In7 : Inport  Port=8
  In8 : Inport  Port=9
  In9 : Inport  Port=10
  In10 : Inport  Port=11
  In11 : Inport  Port=12
  In12 : Inport  Port=13
  In13 : Inport  Port=14
  In14 : Inport  Port=15
  In15 : Inport  Port=16
  In16 : Inport  Port=17
  ch : Inport  Port=18
  r_tone_scale_sel : Inport  Port=19
  AddSub{1..9,27} (10 alike) : xbsIndex_r4/AddSub  mode=Addition  use_carryin=off  use_carryout=off  en=off  latency=3  precision=User Defined  arith_type="Signed  (2's comp)"  n_bits=20  bin_pt=15  quantization=Truncate  overflow=Wrap  use_behavioral_HDL=off  hw_selection=Fabric  pipelined=on  dbl_ovrd=off  block_type=addsub
  AddSub{10..11,15,20} (4 alike) : xbsIndex_r4/AddSub  mode=Addition  use_carryin=off  use_carryout=off  en=off  latency=3  precision=User Defined  arith_type="Signed  (2's comp)"  n_bits=16  bin_pt=15  quantization="Round  (unbiased: +/- Inf)"  overflow=Saturate  use_behavioral_HDL=off  hw_selection=Fabric  pipelined=on  dbl_ovrd=off  block_type=addsub
  AddSub{12..14,26} (4 alike) : xbsIndex_r4/AddSub  mode=Addition  use_carryin=off  use_carryout=off  en=off  latency=3  precision=User Defined  arith_type="Signed  (2's comp)"  n_bits=20  bin_pt=15  quantization=Truncate  overflow=Wrap  use_behavioral_HDL=off  hw_selection=Fabric  pipelined=off  dbl_ovrd=off  block_type=addsub
  Delay : xbsIndex_r4/Delay  rst=off  infoeditControl=Selection of Reset will increase slice count due to use of real FFs and instead of SRLs  en=off  latency=18  reg_retiming=off  dbl_ovrd=off  block_type=delay
  Delay1 : xbsIndex_r4/Delay  rst=off  infoeditControl=Selection of Reset will increase slice count due to use of real FFs and instead of SRLs  en=off  latency=18  reg_retiming=off  dbl_ovrd=off  block_type=delay
  Mux : xbsIndex_r4/Mux  inputs=4  en=off  latency=1  precision=User Defined  arith_type="Signed  (2's comp)"  n_bits=16  bin_pt=15  quantization=Truncate  overflow=Wrap  dbl_ovrd=off  block_type=mux
  Register{,1..15} (16 alike) : xbsIndex_r4/Register  init=0  rst=off  en=off  dbl_ovrd=off  block_type=register
  Scale{,1..5} (6 alike) : xbsIndex_r4/Scale  scale_factor=-1  dbl_ovrd=off  block_type=scale
  valid_o : Outport
  out : Outport  Port=2
  ch_o : Outport  Port=3
  wires:
  AddSub2/1 -> Register/1
  AddSub3/1 -> Register1/1
  AddSub4/1 -> Register2/1
  AddSub5/1 -> Register3/1
  AddSub6/1 -> Register4/1
  AddSub7/1 -> Register5/1
  AddSub12/1 -> Register8/1
  AddSub13/1 -> Register9/1
  AddSub1/1 -> Register12/1
  In1/1 -> AddSub2/1
  AddSub8/1 -> Register6/1
  AddSub9/1 -> Register7/1
  AddSub14/1 -> Register10/1
  AddSub27/1 -> Register13/1
  AddSub26/1 -> Register11/1
  In16/1 -> AddSub9/2
  In15/1 -> AddSub9/1
  In14/1 -> AddSub8/2
  In13/1 -> AddSub8/1
  In12/1 -> AddSub7/2
  In11/1 -> AddSub7/1
  In10/1 -> AddSub6/2
  In9/1 -> AddSub6/1
  In7/1 -> AddSub5/1
  In6/1 -> AddSub4/2
  In5/1 -> AddSub4/1
  In4/1 -> AddSub3/2
  In3/1 -> AddSub3/1
  In2/1 -> AddSub2/2
  In8/1 -> AddSub5/2
  Register/1 -> AddSub12/1
  Register1/1 -> AddSub12/2
  Register2/1 -> AddSub13/1
  Register3/1 -> AddSub13/2
  Register4/1 -> AddSub14/1
  Register5/1 -> AddSub14/2
  Register6/1 -> AddSub26/1
  Register7/1 -> AddSub26/2
  Register8/1 -> AddSub1/1
  Register9/1 -> AddSub1/2
  Register10/1 -> AddSub27/1
  Register11/1 -> AddSub27/2
  Register12/1 -> AddSub15/1, Scale/1
  Register13/1 -> AddSub15/2, Scale1/1
  Register14/1 -> Register15/1
  valid/1 -> Delay/1
  ch/1 -> Delay1/1
  Delay/1 -> valid_o/1
  Delay1/1 -> ch_o/1
  r_tone_scale_sel/1 -> Mux/1
  Scale1/1 -> AddSub11/2, Scale2/1
  Scale2/1 -> AddSub10/2, Scale3/1
  Scale4/1 -> AddSub10/1, Scale5/1
  Scale/1 -> AddSub11/1, Scale4/1
  Scale5/1 -> AddSub20/1
  Scale3/1 -> AddSub20/2
  Register15/1 -> out/1
  AddSub20/1 -> Mux/2
  AddSub10/1 -> Mux/3
  AddSub11/1 -> Mux/4
  AddSub15/1 -> Mux/5
  Mux/1 -> Register14/1
